simulink model "OnBoardMatlabExpo2"  (R2016b)
settings: Solver=FixedStepDiscrete  StartTime=0.0  StopTime=10.0  FixedStep=0.002  RelTol=1e-3
PreLoadFcn:
  | waijung.modelPreload; % Required for working with Waijung Blockset. Do not remove.
InitFcn:
  | cubeparameters
values from neighbouring files (symbols this model uses):
  A = [0 0 0 0 0 0 0 0 0 0 283.190307038 0 ... (36 elements, 6x6)]    [K_lqr_3D.mat]
  C = [1 0 0 0 0 0 0 1 0 0 0 0 ... (36 elements, 6x6)]    [K_lqr_3D.mat]
undefined symbols (not defined in the file or in its folder): CPHA_1Edge, CPOL_Low, Duplex, FirstBit_MSB, Full, Link, LQFP100, ST, STM32F407VG, STM32F4DISCOVERY
libraries: simulink x12, stm32f4_io_lib x5, cube_lib x3, stm32f4_spi_lib x3, stm32f4_device_config_lib x1, BC_USB x1, stm32f4_adc_lib x1
(part 2 of 2)

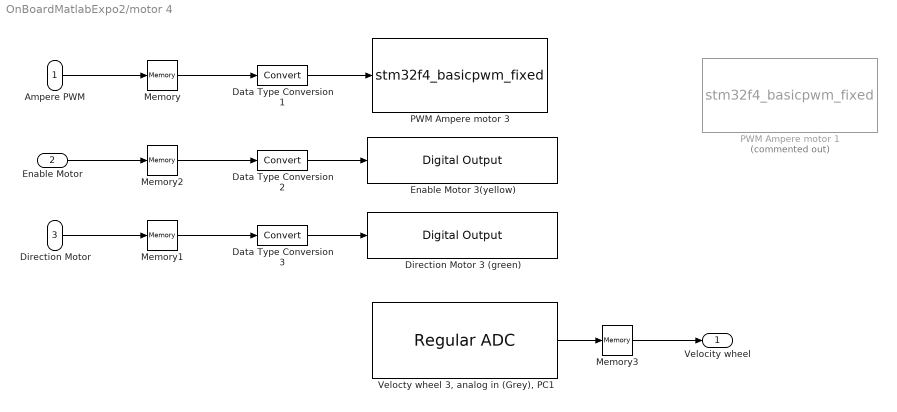
== system OnBoardMatlabExpo2/motor 4 ==
  Ampere PWM : Inport
  Enable Motor : Inport  Port=2
  "Direction Motor " : Inport  Port=3
  Data Type Conversion1 : DataTypeConversion
  Data Type Conversion2 : DataTypeConversion
  Data Type Conversion3 : DataTypeConversion
  Direction Motor 3 (green) : stm32f4_io_lib/Digital Output  use_bitband=on  port=D  speed=100  porttype=Push Pull  porttypestr=PP  use_pin0=off  use_pin1=off  use_pin2=off  use_pin3=off  use_pin4=off  use_pin5=off  use_pin6=off  use_pin7=off  use_pin8=off  use_pin9=off  use_pin10=off  use_pin11=on  use_pin12=off  use_pin13=off  use_pin14=off  use_pin15=off  pinstr=GPIO_Pin_11  usedpinarray="[0  0  0  0  0  0  0  0  0  0  0  1  0  0  0  0]"  bitbandingstr="#define motor4DirectionMotor3green_D11 Peripheral_BB(GPIOD->ODR, 11)  /* Output pin */"  sampletime=-1  sampletimestr=0.002  blockid=motor4DirectionMotor3green  enablecustomportlabel=off  globalinit=off  cinputportlabel=In1, In2  coutputportlabel=0
  Enable Motor 3(yellow) : stm32f4_io_lib/Digital Output  use_bitband=on  port=D  speed=100  porttype=Push Pull  porttypestr=PP  use_pin0=off  use_pin1=off  use_pin2=off  use_pin3=off  use_pin4=off  use_pin5=off  use_pin6=off  use_pin7=off  use_pin8=off  use_pin9=on  use_pin10=off  use_pin11=off  use_pin12=off  use_pin13=off  use_pin14=off  use_pin15=off  pinstr=GPIO_Pin_9  usedpinarray="[0  0  0  0  0  0  0  0  0  1  0  0  0  0  0  0]"  bitbandingstr="#define motor4EnableMotor3yellow_D9 Peripheral_BB(GPIOD->ODR, 9)  /* Output pin */"  sampletime=-1  sampletimestr=0.002  blockid=motor4EnableMotor3yellow  enablecustomportlabel=off  globalinit=off  cinputportlabel=In1, In2  coutputportlabel=0
  Memory{,1..3} (4 alike) : Memory  InheritSampleTime=on
  PWM Ampere motor 1 : S-Function  Commented=on  FunctionName=stm32f4_basicpwm_fixed  Parameters=timer,pwmperiod,uc3m_pwmperiod,ch1pin,ch2pin,ch3pin,ch4pin,sampletime,sampletimestr,blockid,apb,portstr,pinstr,pinmat,timarr,timprescale,chmat,polaritystr  SFunctionDeploymentMode=off  EnableBusSupport=off  mask(stm32f4_basicpwm_fixed){timer=5, pwmperiod=0.02, uc3m_pwmperiod=0.0002, polarity=Active High, polaritystr=TIM_OCPolarity_High, ch1pin=Not available - Do not use, ch2pin=Not available - Do not use, ch3pin=Not available - Do not use, ch4pin=A3, sampletime=0.002, sampletimestr=0.002, blockid=motor3PWMAmperemotor3, portpinstr=,,,A3, enablecustomportlabel=off, cinputportlabel=In1, In2, In3, In4, coutputportlabel=0, callbackgensrccode=off, apb=1, portstr=["A"], pinstr=["GPIO_Pin_3"], pinmat=[1 3], timarr=59999, timprescale=55, chmat=[4]}
      mask prompts: pwmperiod "PWM Period (seconds)"; uc3m_pwmperiod "PWM Signal Period (seconds)"; ch1pin "Channel 1"; ch2pin "Channel 2"; ch3pin "Channel 3"; ch4pin "Channel 4"; sampletime "Sample time (sec)"; sampletimestr "Compiled sample time (sec) in string"; portpinstr "Port pin string"; enablecustomportlabel "Enable custom port labels"; cinputportlabel "Custom input port labels (Ex. In1, In2, In3)"; coutputportlabel "Custom output port labels (Ex. Out1, Out2, Out3)"; callbackgensrccode "Gen source code from callback"; portstr "Port string"; pinstr "Pin string"; pinmat "Pin matrix"; timarr "Timer ARR"; timprescale "Timer PRESCALE"; chmat "Channel order"
      mask help:
      | This block implements basic Edge-aligned Pulse Width Modulation (PWM) generation.
      | All timers are 16-bit. The PWM period is fixed (per timer).
      |
      | This block was fixed by Sr Antonio
      mask init:
      | stm32f4_basicpwm_callback_fixed('init');
      mask Help: web(fullfile(waijungdocroot,'stm32f4_basicpwm.htm'),'-browser')
      mask TypeOptions timer: 1 | 2 | 3 | 4 | 5 | 8 | 9 | 10 | 11 | 12 | 13 | 14
      mask Callback timer: stm32f4_basicpwm_callback_fixed('timer');
      mask Callback pwmperiod: stm32f4_basicpwm_callback_fixed('pwmperiod');
      mask Callback uc3m_pwmperiod: stm32f4_basicpwm_callback_fixed('uc3m_pwmperiod');
      mask TypeOptions polarity: Active High | Active Low
      mask Callback polarity: stm32f4_basicpwm_callback_fixed('polarity');
      mask TypeOptions ch1pin: Not available - Do not use | A0 | A5
      mask Callback ch1pin: stm32f4_basicpwm_callback_fixed('ch1pin');
      mask TypeOptions ch2pin: Not available - Do not use | A1 | B3
      mask Callback ch2pin: stm32f4_basicpwm_callback_fixed('ch2pin');
      mask TypeOptions ch3pin: Not available - Do not use | A2 | B10
      mask Callback ch3pin: stm32f4_basicpwm_callback_fixed('ch3pin');
      mask TypeOptions ch4pin: Not available - Do not use | A3 | B11
      mask Callback ch4pin: stm32f4_basicpwm_callback_fixed('ch4pin');
      mask Callback sampletime: stm32f4_basicpwm_callback_fixed('sampletime');
      mask Callback sampletimestr: stm32f4_basicpwm_callback_fixed('sampletimestr');
      mask Callback blockid: stm32f4_basicpwm_callback_fixed('blockid');
      mask Callback enablecustomportlabel: stm32f4_basicpwm_callback_fixed('enablecustomportlabel')
      mask Display: text(0.95, 0.5, 'UC3M FIXED\nTimer: 5\nPolarity: Active High\nPeriod (sec): 0.0002\nTs (sec): 0.002','ver','middle','hor','right');port_label('input', 1,'CH4 (A3)')
  PWM Ampere motor 3 : S-Function  FunctionName=stm32f4_basicpwm_fixed  Parameters=timer,pwmperiod,uc3m_pwmperiod,ch1pin,ch2pin,ch3pin,ch4pin,sampletime,sampletimestr,blockid,apb,portstr,pinstr,pinmat,timarr,timprescale,chmat,polaritystr  SFunctionDeploymentMode=off  EnableBusSupport=off  mask(stm32f4_basicpwm_fixed){timer=2, pwmperiod=0.02, uc3m_pwmperiod=0.0002, polarity=Active High, polaritystr=TIM_OCPolarity_High, ch1pin=Not available - Do not use, ch2pin=Not available - Do not use, ch3pin=Not available - Do not use, ch4pin=A3, sampletime=0.002, sampletimestr=0.002, blockid=motor4PWMAmperemotor3, portpinstr=,,,A3, enablecustomportlabel=off, cinputportlabel=In1, In2, In3, In4, coutputportlabel=0, callbackgensrccode=off, apb=1, portstr=["A"], pinstr=["GPIO_Pin_3"], pinmat=[1 3], timarr=59999, timprescale=55, chmat=[4]}
      mask prompts: pwmperiod "PWM Period (seconds)"; uc3m_pwmperiod "PWM Signal Period (seconds)"; ch1pin "Channel 1"; ch2pin "Channel 2"; ch3pin "Channel 3"; ch4pin "Channel 4"; sampletime "Sample time (sec)"; sampletimestr "Compiled sample time (sec) in string"; portpinstr "Port pin string"; enablecustomportlabel "Enable custom port labels"; cinputportlabel "Custom input port labels (Ex. In1, In2, In3)"; coutputportlabel "Custom output port labels (Ex. Out1, Out2, Out3)"; callbackgensrccode "Gen source code from callback"; portstr "Port string"; pinstr "Pin string"; pinmat "Pin matrix"; timarr "Timer ARR"; timprescale "Timer PRESCALE"; chmat "Channel order"
      mask help:
      | This block implements basic Edge-aligned Pulse Width Modulation (PWM) generation.
      | All timers are 16-bit. The PWM period is fixed (per timer).
      |
      | This block was fixed by Sr Antonio
      mask init:
      | stm32f4_basicpwm_callback_fixed('init');
      mask Help: web(fullfile(waijungdocroot,'stm32f4_basicpwm.htm'),'-browser')
      mask TypeOptions timer: 1 | 2 | 3 | 4 | 5 | 8 | 9 | 10 | 11 | 12 | 13 | 14
      mask Callback timer: stm32f4_basicpwm_callback_fixed('timer');
      mask Callback pwmperiod: stm32f4_basicpwm_callback_fixed('pwmperiod');
      mask Callback uc3m_pwmperiod: stm32f4_basicpwm_callback_fixed('uc3m_pwmperiod');
      mask TypeOptions polarity: Active High | Active Low
      mask Callback polarity: stm32f4_basicpwm_callback_fixed('polarity');
      mask TypeOptions ch1pin: Not available - Do not use | A0 | A5
      mask Callback ch1pin: stm32f4_basicpwm_callback_fixed('ch1pin');
      mask TypeOptions ch2pin: Not available - Do not use | A1 | B3
      mask Callback ch2pin: stm32f4_basicpwm_callback_fixed('ch2pin');
      mask TypeOptions ch3pin: Not available - Do not use | A2 | B10
      mask Callback ch3pin: stm32f4_basicpwm_callback_fixed('ch3pin');
      mask TypeOptions ch4pin: Not available - Do not use | A3 | B11
      mask Callback ch4pin: stm32f4_basicpwm_callback_fixed('ch4pin');
      mask Callback sampletime: stm32f4_basicpwm_callback_fixed('sampletime');
      mask Callback sampletimestr: stm32f4_basicpwm_callback_fixed('sampletimestr');
      mask Callback blockid: stm32f4_basicpwm_callback_fixed('blockid');
      mask Callback enablecustomportlabel: stm32f4_basicpwm_callback_fixed('enablecustomportlabel')
      mask Display: text(0.95, 0.5, 'UC3M FIXED\nTimer: 2\nPolarity: Active High\nPeriod (sec): 0.0002\nTs (sec): 0.002','ver','middle','hor','right');port_label('input', 1,'CH4 (A3)')
  "Velocty wheel 3, analog in (Grey), PC1" : stm32f4_adc_lib/Regular ADC  adcmodule=3  outputdatatype=Double  prescaler=2  prescalerstr=ADC_Prescaler_Div2  chsamplingtime=Auto  chsamplingtimestr=ADC_SampleTime_480Cycles  read_an0=off  read_an1=off  read_an2=off  read_an3=off  read_an4=off  read_an5=off  read_an6=off  read_an7=off  read_an8=off  read_an9=off  read_an10=off  read_an11=on  read_an12=off  read_an13=off  read_an14=off  read_an15=off  read_an16=off  read_an17=off  read_an18=off  pinstr=GPIO_Pin_11  usedpinarray="[0  0  0  0  0  0  0  0  0  0  0  1  0  0  0  0  0  0  0]"  usedportidarray=[2]  usedpinidarray=[1]  usedpinidcount=1  sampletime=0.002  blockid=motor4Veloctywheel3analoginGreyPC1  enablecustomportlabel=off  cinputportlabel=0  coutputportlabel=Out1, Out2
  Velocity wheel : Outport
  wires:
  Ampere PWM/1 -> Memory/1
  Data Type Conversion3/1 -> Direction Motor 3 (green)/1
  Data Type Conversion2/1 -> Enable Motor 3(yellow)/1
  Memory/1 -> Data Type Conversion1/1
  Memory2/1 -> Data Type Conversion2/1
  "Direction Motor "/1 -> Memory1/1
  Memory1/1 -> Data Type Conversion3/1
  Enable Motor/1 -> Memory2/1
  "Velocty wheel 3, analog in (Grey), PC1"/1 -> Memory3/1
  Memory3/1 -> Velocity wheel/1
  Data Type Conversion1/1 -> PWM Ampere motor 3/1

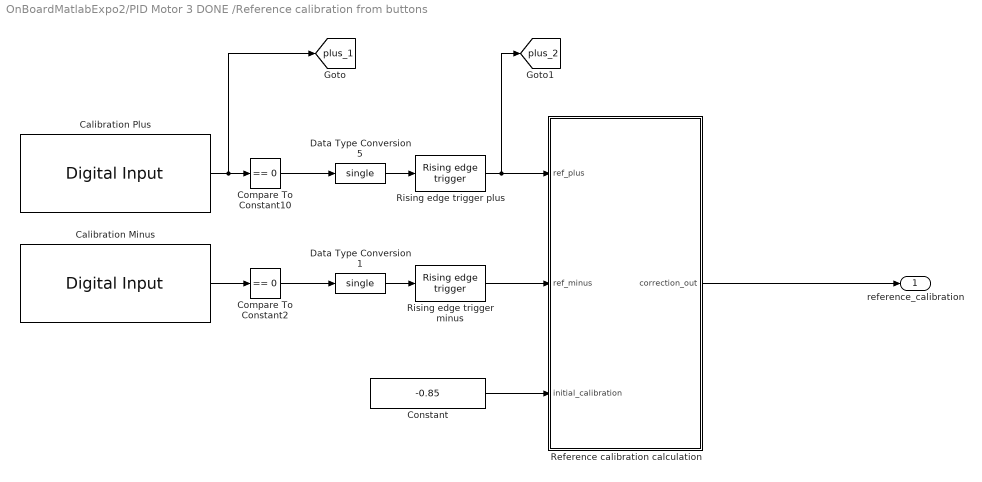
== system OnBoardMatlabExpo2/PID Motor 3 DONE /Reference calibration from buttons ==
  Calibration Minus : stm32f4_io_lib/Digital Input  port=E  speed=100  porttype=Pull Up  porttypestr=UP  use_pin0=off  use_pin1=off  use_pin2=off  use_pin3=off  use_pin4=off  use_pin5=off  use_pin6=off  use_pin7=off  use_pin8=off  use_pin9=off  use_pin10=off  use_pin11=off  use_pin12=off  use_pin13=off  use_pin14=on  use_pin15=off  pinstr=GPIO_Pin_14  usedpinarray="[0  0  0  0  0  0  0  0  0  0  0  0  0  0  1  0]"  bitbandingstr="#define PIDMotor3DONEReferencecalibrationfrombuttonsCalibrationMinus_E14 Peripheral_BB(GPIOE->IDR, 14)  /* Output pin */"  sampletime=0.002  sampletimestr=0.002  blockid=PIDMotor3DONEReferencecalibrationfrombuttonsCalibrationMinus  enablecustomportlabel=off  glabalinit=off  cinputportlabel=In1, In2  coutputportlabel=Out1, Out2
  Calibration Plus : stm32f4_io_lib/Digital Input  port=E  speed=100  porttype=Pull Up  porttypestr=UP  use_pin0=off  use_pin1=off  use_pin2=off  use_pin3=off  use_pin4=off  use_pin5=off  use_pin6=off  use_pin7=off  use_pin8=off  use_pin9=off  use_pin10=off  use_pin11=on  use_pin12=off  use_pin13=off  use_pin14=off  use_pin15=off  pinstr=GPIO_Pin_11  usedpinarray="[0  0  0  0  0  0  0  0  0  0  0  1  0  0  0  0]"  bitbandingstr="#define PIDMotor3DONEReferencecalibrationfrombuttonsCalibrationPlus_E11 Peripheral_BB(GPIOE->IDR, 11)  /* Output pin */"  sampletime=0.002  sampletimestr=0.002  blockid=PIDMotor3DONEReferencecalibrationfrombuttonsCalibrationPlus  enablecustomportlabel=off  glabalinit=off  cinputportlabel=In1, In2  coutputportlabel=Out1, Out2
  Compare To Constant10 : simulink/Logic and Bit Operations/Compare To Constant  relop===  const=0  OutDataTypeStr=boolean  ZeroCross=off
  Compare To Constant2 : simulink/Logic and Bit Operations/Compare To Constant  relop===  const=0  OutDataTypeStr=boolean  ZeroCross=off
  Constant : Constant  Value=-0.85
  Data Type Conversion1 : DataTypeConversion  OutDataTypeStr=single
  Data Type Conversion5 : DataTypeConversion  OutDataTypeStr=single
  Reference calibration calculation : MATLAB Function  TreatAsAtomicUnit=on
  Rising edge trigger minus : cube_lib/Rising edge trigger
  Rising edge trigger plus : cube_lib/Rising edge trigger
  reference_calibration : Outport
  tag scope: plus_1=global, plus_2=global
  wires:
  Data Type Conversion5/1 -> Rising edge trigger plus/1
  Reference calibration calculation/1(correction_out) -> reference_calibration/1
  Calibration Minus/1 -> Compare To Constant2/1
  Compare To Constant10/1 -> Data Type Conversion5/1
  Compare To Constant2/1 -> Data Type Conversion1/1
  Calibration Plus/1 -> [plus_1], Compare To Constant10/1
  Rising edge trigger minus/1 -> Reference calibration calculation/2(ref_minus)
  Data Type Conversion1/1 -> Rising edge trigger minus/1
  Rising edge trigger plus/1 -> [plus_2], Reference calibration calculation/1(ref_plus)
  Constant/1 -> Reference calibration calculation/3(initial_calibration)

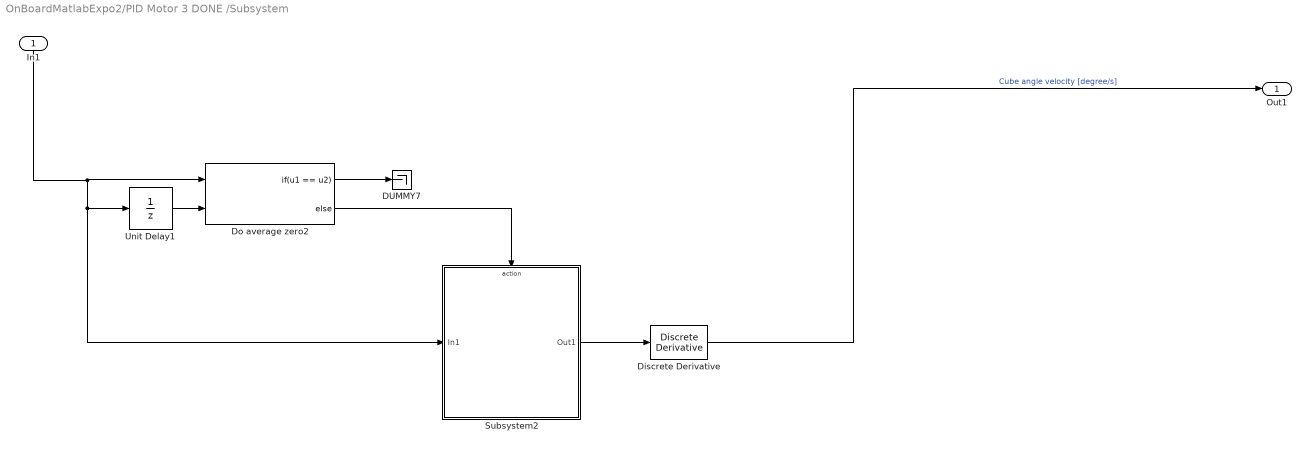
== system OnBoardMatlabExpo2/PID Motor 3 DONE /Subsystem ==
  In1 : Inport
  DUMMY7 : Terminator
  Discrete Derivative : simulink/Discrete/Discrete Derivative  gainval=1.0  ICPrevScaledInput=0.0  InputProcessing=Inherited  OutMin=[]  OutMax=[]  OutDataType=fixdt(1, 16)  OutScaling=2^-10  DoSatur=off
  Do average zero2 : If  NumInputs=2  IfExpression=u1 == u2
  Subsystem2 : Subsystem
  Unit Delay1 : UnitDelay  SampleTime=-1
  Out1 : Outport
  wires:
  Do average zero2/2 -> Subsystem2/Action
  Unit Delay1/1 -> Do average zero2/2
  Discrete Derivative/1 -> Out1/1  "Cube angle velocity [degree/s]"
  Subsystem2/1(Out1) -> Discrete Derivative/1
  In1/1 -> Subsystem2/1(In1), Unit Delay1/1, Do average zero2/1
  Do average zero2/1 -> DUMMY7/1

== system OnBoardMatlabExpo2/PID Motor 3 DONE /Subsystem2 ==
  In1 : Inport
  DUMMY7 : Terminator
  Do average zero1 : If  NumInputs=2  IfExpression=u1 == u2
  Subsystem1 : Subsystem
  Unit Delay3 : UnitDelay  SampleTime=-1
  Out2 : Outport
  wires:
  Unit Delay3/1 -> Do average zero1/2
  Do average zero1/2 -> Subsystem1/Action
  In1/1 -> Subsystem1/1(In1), Unit Delay3/1, Do average zero1/1
  Subsystem1/1(Out1) -> Out2/1
  Do average zero1/1 -> DUMMY7/1

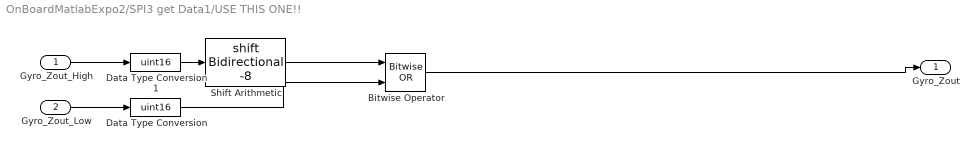
== system OnBoardMatlabExpo2/SPI3 get Data1/USE THIS ONE!! ==
  "Gyro_Zout_High " : Inport
  Gyro_Zout_Low : Inport  Port=2
  Bitwise Operator : simulink/Logic and Bit Operations/Bitwise Operator  logicop=OR  UseBitMask=off  NumInputPorts=2  BitMask=bin2dec('11011001')  BitMaskRealWorld=Stored Integer
  Data Type Conversion : DataTypeConversion  OutDataTypeStr=uint16
  Data Type Conversion1 : DataTypeConversion  OutDataTypeStr=uint16
  Shift Arithmetic : ArithShift  BitShiftNumber=-8
  Gyro_Zout : Outport
  wires:
  Gyro_Zout_Low/1 -> Data Type Conversion/1
  "Gyro_Zout_High "/1 -> Data Type Conversion1/1
  Data Type Conversion1/1 -> Shift Arithmetic/1
  Data Type Conversion/1 -> Bitwise Operator/2
  Shift Arithmetic/1 -> Bitwise Operator/1
  Bitwise Operator/1 -> Gyro_Zout/1

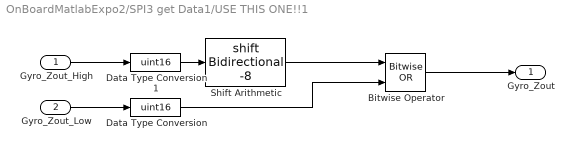
== system OnBoardMatlabExpo2/SPI3 get Data1/USE THIS ONE!!1 ==
  "Gyro_Zout_High " : Inport
  Gyro_Zout_Low : Inport  Port=2
  Bitwise Operator : simulink/Logic and Bit Operations/Bitwise Operator  logicop=OR  UseBitMask=off  NumInputPorts=2  BitMask=bin2dec('11011001')  BitMaskRealWorld=Stored Integer
  Data Type Conversion : DataTypeConversion  OutDataTypeStr=uint16
  Data Type Conversion1 : DataTypeConversion  OutDataTypeStr=uint16
  Shift Arithmetic : ArithShift  BitShiftNumber=-8
  Gyro_Zout : Outport
  wires:
  Gyro_Zout_Low/1 -> Data Type Conversion/1
  "Gyro_Zout_High "/1 -> Data Type Conversion1/1
  Data Type Conversion1/1 -> Shift Arithmetic/1
  Data Type Conversion/1 -> Bitwise Operator/2
  Shift Arithmetic/1 -> Bitwise Operator/1
  Bitwise Operator/1 -> Gyro_Zout/1

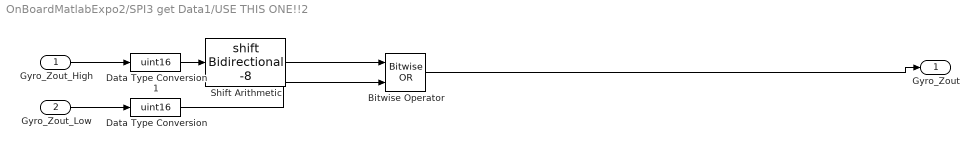
== system OnBoardMatlabExpo2/SPI3 get Data1/USE THIS ONE!!2 ==
  "Gyro_Zout_High " : Inport
  Gyro_Zout_Low : Inport  Port=2
  Bitwise Operator : simulink/Logic and Bit Operations/Bitwise Operator  logicop=OR  UseBitMask=off  NumInputPorts=2  BitMask=bin2dec('11011001')  BitMaskRealWorld=Stored Integer
  Data Type Conversion : DataTypeConversion  OutDataTypeStr=uint16
  Data Type Conversion1 : DataTypeConversion  OutDataTypeStr=uint16
  Shift Arithmetic : ArithShift  BitShiftNumber=-8
  Gyro_Zout : Outport
  wires:
  Gyro_Zout_Low/1 -> Data Type Conversion/1
  "Gyro_Zout_High "/1 -> Data Type Conversion1/1
  Data Type Conversion1/1 -> Shift Arithmetic/1
  Data Type Conversion/1 -> Bitwise Operator/2
  Shift Arithmetic/1 -> Bitwise Operator/1
  Bitwise Operator/1 -> Gyro_Zout/1

== system OnBoardMatlabExpo2/PID Motor 3 DONE /Subsystem/Subsystem2 ==
  In1 : Inport
  Action Port : ActionPort  ActionType=else
  Subsystem : Subsystem
  Unit Delay1 : UnitDelay  SampleTime=-1
  Out1 : Outport
  wires:
  In1/1 -> Subsystem/1(In1)
  Subsystem/1(Average Speed) -> Out1/1  "Speed, PA1"
  Subsystem/2(One old Speed) -> Unit Delay1/1
  Unit Delay1/1 -> Subsystem/2(One old speed)

== system OnBoardMatlabExpo2/PID Motor 3 DONE /Subsystem2/Subsystem1 ==
  In1 : Inport
  Action Port : ActionPort  ActionType=else
  Subsystem : Subsystem
  Unit Delay1 : UnitDelay  SampleTime=-1
  Out1 : Outport
  wires:
  In1/1 -> Subsystem/1(In1)
  Subsystem/1(Average Speed) -> Out1/1  "Speed, PA1"
  Subsystem/2(One old Speed) -> Unit Delay1/1
  Unit Delay1/1 -> Subsystem/2(One old speed)

== system OnBoardMatlabExpo2/PID Motor 3 DONE /Subsystem/Subsystem2/Subsystem ==
  In1 : Inport
  One old speed : Inport  Port=2
  Add2 : Sum
  Gain2 : Gain  Gain=0.5
  Gain3 : Gain  Gain=0.5
  Average Speed : Outport
  One old Speed : Outport  Port=2
  wires:
  Add2/1 -> One old Speed/1, Average Speed/1  "Speed, PA1"
  One old speed/1 -> Gain2/1
  In1/1 -> Gain3/1
  Gain2/1 -> Add2/2
  Gain3/1 -> Add2/1

== system OnBoardMatlabExpo2/PID Motor 3 DONE /Subsystem2/Subsystem1/Subsystem ==
  In1 : Inport
  One old speed : Inport  Port=2
  Add2 : Sum
  Gain2 : Gain  Gain=0.3
  Gain3 : Gain  Gain=0.7
  Average Speed : Outport
  One old Speed : Outport  Port=2
  wires:
  Add2/1 -> One old Speed/1, Average Speed/1  "Speed, PA1"
  One old speed/1 -> Gain2/1
  In1/1 -> Gain3/1
  Gain2/1 -> Add2/2
  Gain3/1 -> Add2/1

== matlab function OnBoardMatlabExpo2/USB VCP Send/Sample counter ==
  data: sample output
function sample = SampleCounter
%#codegen

persistent sample_count;

if isempty(sample_count)
    sample_count = 0;
end

sample_count = sample_count + 1;

sample = sample_count;

== matlab function OnBoardMatlabExpo2/PID Motor 3 DONE /Reference calibration from buttons/Reference calibration calculation ==
  data: ref_plus input; correction_out output; ref_minus input; initial_calibration input
function correction_out = ReferenceCalibration(ref_plus,ref_minus,initial_calibration)
%#codegen

persistent correction;

delta_correction = 0.05; % NOTE: Degrees!

if isempty(correction)
    correction = initial_calibration;   % Initial calibration is estimated center of gravity offset from geometrical center, in degrees.
end

if ref_plus == 1
    correction = correction + delta_correction;
end

if ref_minus == 1
    correction = correction - delta_correction;
end

correction_out = correction;

== matlab function OnBoardMatlabExpo2/SPI3 get Data1/Take away Sensor fail reading ==
  data: y output; new input; old input
function y = fcn(new, old)
%#codegen
if(new > -257 && new < -200)
   y = old;
else
    y = new;
end

== matlab function OnBoardMatlabExpo2/SPI3 get Data1/Take away Sensor fail reading if two bad in raw ==
  data: y output; new input; old input
function y = fcn(new, old)
%#codegen
if(new > -257 && new < -200)
   y = old;
else
    y = new;
end
